simulink model "PID_lab4"  (R2014a)
settings: Solver=ode45  StartTime=0.0  StopTime=40  RelTol=1e-3
libraries: simulink x1
settings Model: Creator=Omar Emad  LastModifiedBy=Omar Emad

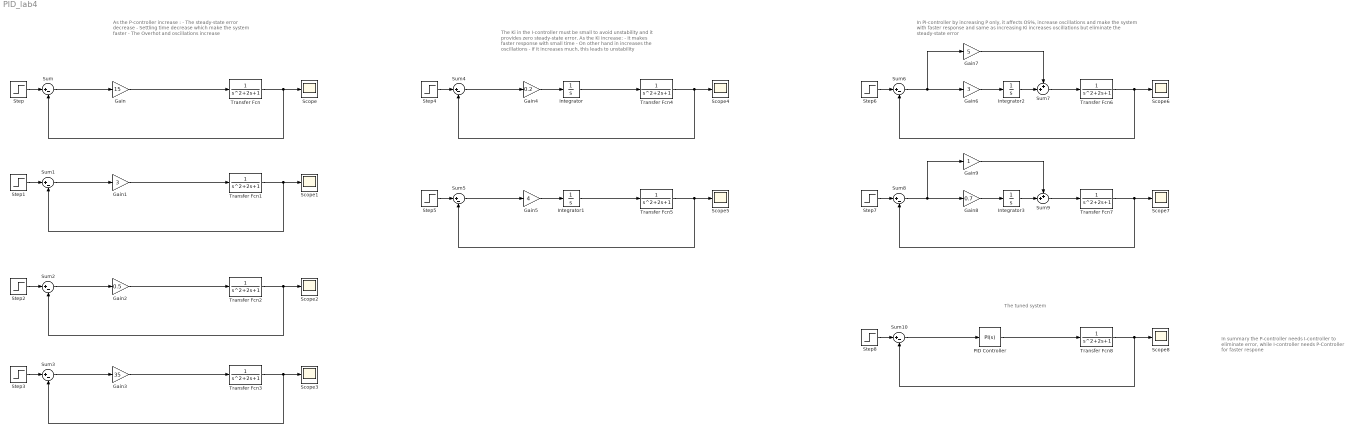
== system PID_lab4 ==
  note: In summary the P-controller needs
      | I-controller to eliminate error, while
      | I-controller needs P-Controller for faster respone
  note: The tuned system
  note: In PI-controller by increasing P only, it affects OS%, increase oscillations
      | and make the system with faster response
      | and same as increasing Ki increases oscillations but eliminate the steady-state error
  note: The Ki in the I-controller must be small to avoid unstability
      | and it provides zero steady-state error. As the Ki increase:
      | - It makes faster response with small time
      | - On other hand in increases the oscillations
      | - If it increases much, this leads to unstability
  note: As the P-controller increase :
      | -  The steady-state error decrease
      | - Settling time decrease which make the system faster
      | - The Overhot and oscillations increase
  Gain : Gain  Gain=15
  Gain1 : Gain  Gain=3
  Gain2 : Gain  Gain=0.5
  Gain3 : Gain  Gain=35
  Gain4 : Gain  Gain=0.2
  Gain5 : Gain  Gain=4
  Gain6 : Gain  Gain=3
  Gain7 : Gain  Gain=5
  Gain8 : Gain  Gain=0.7
  Gain9 : Gain
  Integrator{,1..3} (4 alike) : Integrator
  PID Controller : simulink/Continuous/PID Controller  Controller=PI  TimeDomain=Continuous-time  SampleTime=1  IntegratorMethod=Forward Euler  FilterMethod=Forward Euler  Form=Parallel  P=0.761311081419729  I=0.475488409080512  D=0  N=100  InitialConditionSource=internal  InitialConditionForIntegrator=0  InitialConditionForFilter=0  ExternalReset=none  LimitOutput=off  UpperSaturationLimit=inf  LowerSaturationLimit=-inf  LinearizeAsGain=on  AntiWindupMode=none  Kb=1  TrackingMode=off  Kt=1  PParamMin=[]  PParamMax=[]  IParamMin=[]  IParamMax=[]  DParamMin=[]  DParamMax=[]  NParamMin=[]  NParamMax=[]  KbParamMin=[]  KbParamMax=[]  KtParamMin=[]  KtParamMax=[]  POutMin=[]  POutMax=[]  IOutMin=[]  IOutMax=[]  DOutMin=[]  DOutMax=[]  NOutMin=[]  NOutMax=[]  KbOutMin=[]  KbOutMax=[]  KtOutMin=[]  KtOutMax=[]  IntegratorOutMin=[]  IntegratorOutMax=[]  FilterOutMin=[]  FilterOutMax=[]  SumOutMin=[]  SumOutMax=[]  SumI1OutMin=[]  SumI1OutMax=[]  SumI2OutMin=[]  SumI2OutMax=[]  SumI3OutMin=[]  SumI3OutMax=[]  SumDOutMin=[]  SumDOutMax=[]  SaturationOutMin=[]  SaturationOutMax=[]  IntegratorContinuousStateAttributes=''  IntegratorStateMustResolveToSignalObject=off  IntegratorRTWStateStorageClass=Auto  FilterContinuousStateAttributes=''  FilterStateMustResolveToSignalObject=off  FilterRTWStateStorageClass=Auto
  Scope{,1..8} (9 alike) : Scope
      Scope2 settings: SaveName=ScopeData2
      Scope3 settings: SaveName=ScopeData3
      Scope4 settings: SaveName=ScopeData4
      Scope5 settings: SaveName=ScopeData5
      Scope6 settings: SaveName=ScopeData6
      Scope7 settings: SaveName=ScopeData7
      Scope8 settings: SaveName=ScopeData8
  Step{,1..8} (9 alike) : Step  SampleTime=0
  Sum{,1..6,8,10} (9 alike) : Sum  Inputs=|+-
  Sum7 : Sum  Inputs=++|
  Sum9 : Sum  Inputs=++|
  Transfer Fcn{,1..8} (9 alike) : TransferFcn
  wires:
  Gain/1 -> Transfer Fcn/1
  Step/1 -> Sum/1
  Sum/1 -> Gain/1
  Transfer Fcn/1 -> Sum/2, Scope/1
  Gain1/1 -> Transfer Fcn1/1
  Step1/1 -> Sum1/1
  Sum1/1 -> Gain1/1
  Transfer Fcn1/1 -> Scope1/1, Sum1/2
  Gain2/1 -> Transfer Fcn2/1
  Step2/1 -> Sum2/1
  Sum2/1 -> Gain2/1
  Transfer Fcn2/1 -> Sum2/2, Scope2/1
  Gain3/1 -> Transfer Fcn3/1
  Step3/1 -> Sum3/1
  Sum3/1 -> Gain3/1
  Transfer Fcn3/1 -> Scope3/1, Sum3/2
  Gain4/1 -> Integrator/1
  Step4/1 -> Sum4/1
  Sum4/1 -> Gain4/1
  Transfer Fcn4/1 -> Sum4/2, Scope4/1
  Integrator/1 -> Transfer Fcn4/1
  Gain5/1 -> Integrator1/1
  Step5/1 -> Sum5/1
  Sum5/1 -> Gain5/1
  Transfer Fcn5/1 -> Scope5/1, Sum5/2
  Integrator1/1 -> Transfer Fcn5/1
  Gain6/1 -> Integrator2/1
  Step6/1 -> Sum6/1
  Sum6/1 -> Gain7/1, Gain6/1
  Transfer Fcn6/1 -> Scope6/1, Sum6/2
  Integrator2/1 -> Sum7/2
  Sum7/1 -> Transfer Fcn6/1
  Gain7/1 -> Sum7/1
  Gain8/1 -> Integrator3/1
  Step7/1 -> Sum8/1
  Sum8/1 -> Gain8/1, Gain9/1
  Transfer Fcn7/1 -> Sum8/2, Scope7/1
  Integrator3/1 -> Sum9/2
  Sum9/1 -> Transfer Fcn7/1
  Gain9/1 -> Sum9/1
  Step8/1 -> Sum10/1
  Transfer Fcn8/1 -> Sum10/2, Scope8/1
  Sum10/1 -> PID Controller/1
  PID Controller/1 -> Transfer Fcn8/1
